simulink model "understanding_ofDataInportExport"  (R2024b)
settings: Solver=VariableStepAuto  StartTime=0.0  StopTime=10  MaxStep=0.01  RelTol=1e-3
values from neighbouring files (symbols this model uses):
  k = input(prompt)    [understanding_script_ofDataInportExport.m]
settings Model: Creator=admin  LastModifiedBy=admin

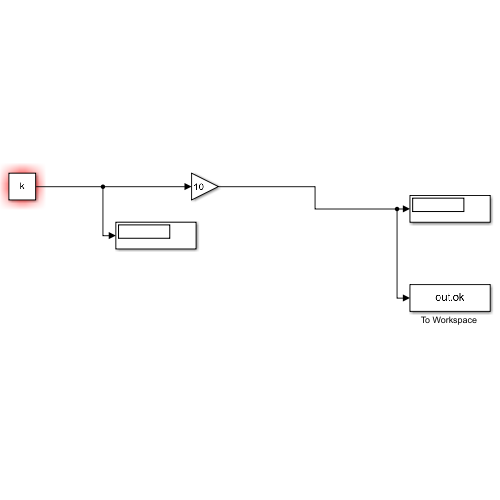
[thumbnail: Simulink's stored preview of the top-level diagram]
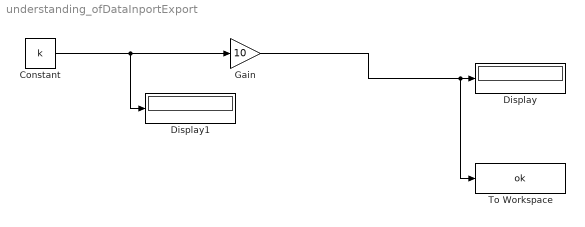
== system understanding_ofDataInportExport ==
  Constant : Constant  Value=k
  Display : Display
  Display1 : Display
  Gain : Gain  Gain=10
  "To Workspace " : ToWorkspace  VariableName=ok  SampleTime=-1
  wires:
  Constant/1 -> Display1/1, Gain/1
  Gain/1 -> "To Workspace "/1, Display/1
